simulink model "Quest"  (R2024b)
settings: Solver=VariableStepAuto  StartTime=0.0  StopTime=10.0  RelTol=1e-3
libraries: matrix_library x2
settings Model: Creator=parrot  LastModifiedBy=parrot

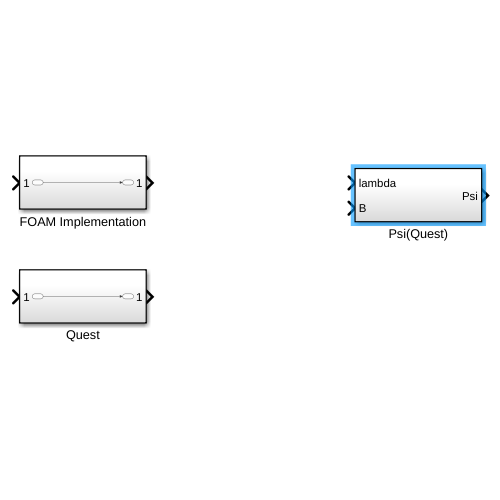
[thumbnail: Simulink's stored preview of the top-level diagram]
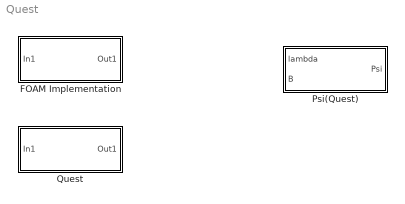
== system Quest ==
  FOAM Implementation : Subsystem
  Psi(Quest) : Subsystem
  Quest : Subsystem

== system Quest/FOAM Implementation ==
  In1 : Inport
  Out1 : Outport
  wires:
  In1/1 -> Out1/1

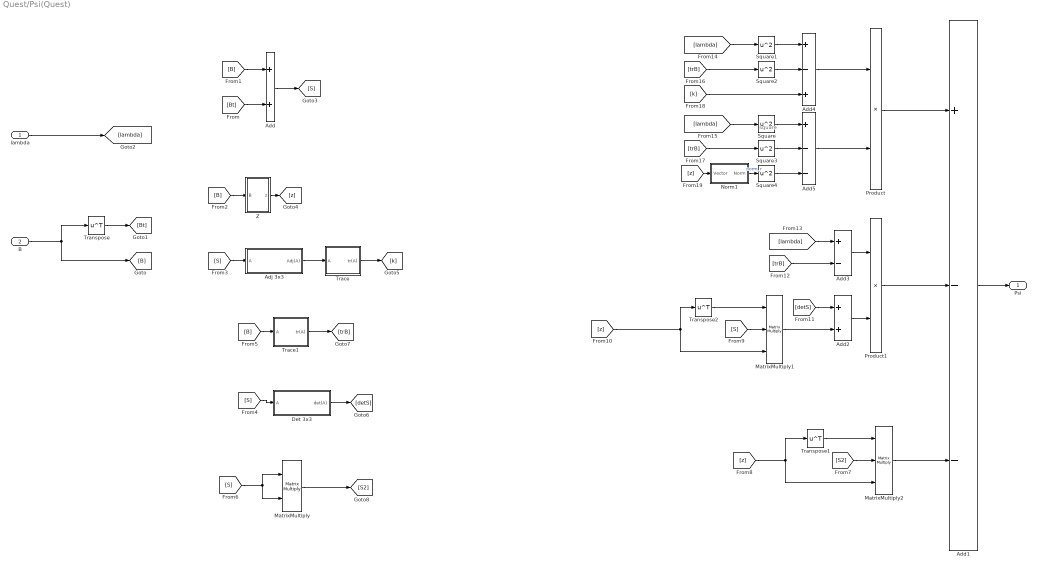
== system Quest/Psi(Quest) ==
  note: square
  lambda : Inport
  B : Inport  Port=2
  Add : Sum
  Add1 : Sum  Inputs=+--
  Add2 : Sum
  Add3 : Sum  Inputs=+-
  Add4 : Sum  Inputs=+-+
  Add5 : Sum  Inputs=+--
  Adj 3x3 : Subsystem
  Det 3x3 : Subsystem
  MatrixMultiply : Product  Multiplication=Matrix(*)
  MatrixMultiply1 : Product  Inputs=3  Multiplication=Matrix(*)
  MatrixMultiply2 : Product  Inputs=3  Multiplication=Matrix(*)
  Norm1 : Subsystem
  Product : Product
  Product1 : Product
  Square{,1..4} (5 alike) : Math  Operator=square
  Trace : Subsystem
  Trace1 : Subsystem
  Transpose : Math  Operator=transpose
  Transpose1 : Math  Operator=transpose
  Transpose2 : Math  Operator=transpose
  Z : Subsystem
  Psi : Outport
  wires:
  Transpose/1 -> [Bt]
  B/1 -> Transpose/1, [B]
  lambda/1 -> [lambda]
  Add/1 -> [S]
  [B] -> Add/1
  [Bt] -> Add/2
  Z/1(z) -> [z]
  [B] -> Z/1(B)
  Adj 3x3/1(Adj(A)) -> Trace/1(A)
  Trace/1(tr(A)) -> [k]
  [S] -> Adj 3x3/1(A)
  [S] -> Det 3x3/1(A)
  Det 3x3/1(det(A)) -> [detS]
  [B] -> Trace1/1(A)
  Trace1/1(tr(A)) -> [trB]
  Add1/1 -> Psi/1
  Product/1 -> Add1/1
  Product1/1 -> Add1/2
  [S] -> MatrixMultiply/1, MatrixMultiply/2
  MatrixMultiply/1 -> [S2]
  MatrixMultiply2/1 -> Add1/3
  [S2] -> MatrixMultiply2/2
  Transpose1/1 -> MatrixMultiply2/1
  [z] -> MatrixMultiply2/3, Transpose1/1
  Transpose2/1 -> MatrixMultiply1/1
  [S] -> MatrixMultiply1/2
  [z] -> MatrixMultiply1/3, Transpose2/1
  Add2/1 -> Product1/2
  MatrixMultiply1/1 -> Add2/2
  [detS] -> Add2/1
  Add3/1 -> Product1/1
  [trB] -> Add3/2
  [lambda] -> Add3/1
  Add4/1 -> Product/1
  Add5/1 -> Product/2
  Square/1 -> Add5/1
  Square1/1 -> Add4/1
  [lambda] -> Square1/1
  [lambda] -> Square/1
  Square2/1 -> Add4/2
  Square3/1 -> Add5/2
  [trB] -> Square2/1
  [trB] -> Square3/1
  Square4/1 -> Add5/3
  [k] -> Add4/3
  Norm1/1(Norm) -> Square4/1  "norm_r"
  [z] -> Norm1/1(Vector)

== system Quest/Quest ==
  In1 : Inport
  Out1 : Outport
  wires:
  In1/1 -> Out1/1

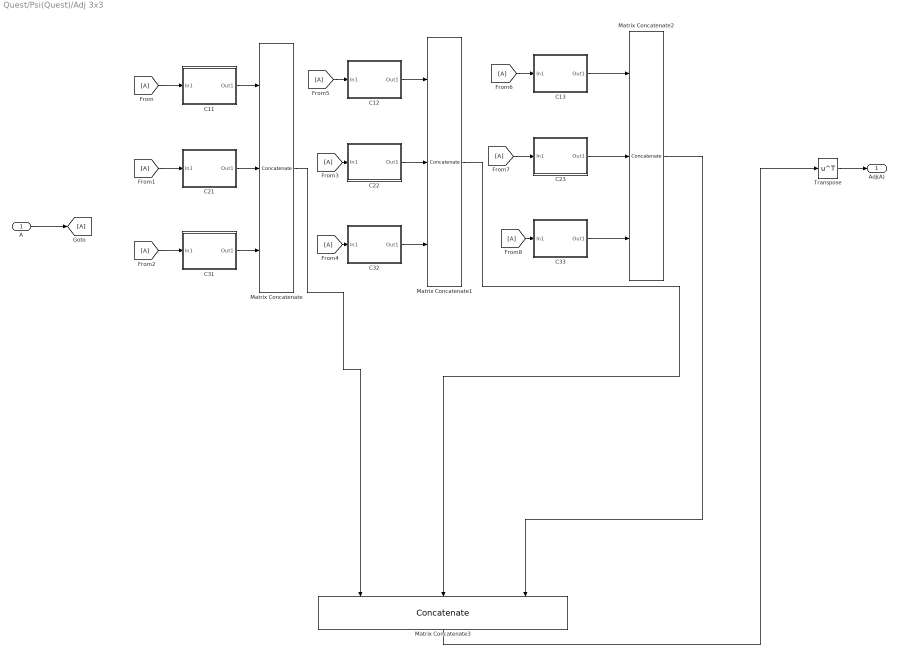
== system Quest/Psi(Quest)/Adj 3x3 ==
  A : Inport
  C11 : Subsystem
  C12 : Subsystem
  C13 : Subsystem
  C21 : Subsystem
  C22 : Subsystem
  C23 : Subsystem
  C31 : Subsystem
  C32 : Subsystem
  C33 : Subsystem
  From{,1..8} (9 alike) : From
  Goto : Goto
  Matrix Concatenate : Concatenate  NumInputs=3  Mode=Multidimensional array
  Matrix Concatenate1 : Concatenate  NumInputs=3  Mode=Multidimensional array
  Matrix Concatenate2 : Concatenate  NumInputs=3  Mode=Multidimensional array
  Matrix Concatenate3 : Concatenate  NumInputs=3  Mode=Multidimensional array  ConcatenateDimension=2
  Transpose : Math  Operator=transpose
  Adj(A) : Outport
  wires:
  Transpose/1 -> Adj(A)/1
  A/1 -> Goto/1
  C11/1(Out1) -> Matrix Concatenate/1
  C21/1(Out1) -> Matrix Concatenate/2
  C31/1(Out1) -> Matrix Concatenate/3
  C22/1(Out1) -> Matrix Concatenate1/2
  C12/1(Out1) -> Matrix Concatenate1/1
  C32/1(Out1) -> Matrix Concatenate1/3
  C23/1(Out1) -> Matrix Concatenate2/2
  C13/1(Out1) -> Matrix Concatenate2/1
  C33/1(Out1) -> Matrix Concatenate2/3
  Matrix Concatenate3/1 -> Transpose/1
  Matrix Concatenate2/1 -> Matrix Concatenate3/3
  Matrix Concatenate1/1 -> Matrix Concatenate3/2
  Matrix Concatenate/1 -> Matrix Concatenate3/1
  From/1 -> C11/1(In1)
  From1/1 -> C21/1(In1)
  From2/1 -> C31/1(In1)
  From3/1 -> C22/1(In1)
  From4/1 -> C32/1(In1)
  From5/1 -> C12/1(In1)
  From6/1 -> C13/1(In1)
  From7/1 -> C23/1(In1)
  From8/1 -> C33/1(In1)

== system Quest/Psi(Quest)/Det 3x3 ==
  A : Inport
  Adj 3x3 : Subsystem
  Matrix Multiply : Product  Multiplication=Matrix(*)
  Selector : Selector  NumberOfDimensions=2  InputPortWidth=3  IndexOptions=Index vector (dialog),Index vector (dialog)  Indices=1,1  OutputSizes=1,1
  det(A) : Outport
  wires:
  A/1 -> Adj 3x3/1(In1), Matrix Multiply/1
  Adj 3x3/1(Out1) -> Matrix Multiply/2
  Matrix Multiply/1 -> Selector/1
  Selector/1 -> det(A)/1

== system Quest/Psi(Quest)/Norm1 ==
  Vector : Inport
  Add : Sum  Inputs=+++
  Demux : Demux  Outputs=3
  Sqrt : Sqrt
  Square : Math  Operator=square
  Square1 : Math  Operator=square
  Square2 : Math  Operator=square
  Norm : Outport
  wires:
  Square/1 -> Add/1
  Add/1 -> Sqrt/1
  Demux/3 -> Square1/1
  Square2/1 -> Add/2
  Square1/1 -> Add/3
  Demux/1 -> Square/1
  Demux/2 -> Square2/1
  Vector/1 -> Demux/1
  Sqrt/1 -> Norm/1

== system Quest/Psi(Quest)/Trace ==
  A : Inport
  Extract Diagonal : matrix_library/Extract Diagonal
      settings: LibrarySourceBlock=|
      | simulink/Matrix
      | Operations/Extract Diagonal
  Sum of Elements : Sum  Inputs=+
  tr(A) : Outport
  wires:
  A/1 -> Extract Diagonal/1
  Extract Diagonal/1 -> Sum of Elements/1
  Sum of Elements/1 -> tr(A)/1

== system Quest/Psi(Quest)/Trace1 ==
  A : Inport
  Extract Diagonal : matrix_library/Extract Diagonal
  Sum of Elements : Sum  Inputs=+
  tr(A) : Outport
  wires:
  A/1 -> Extract Diagonal/1
  Extract Diagonal/1 -> Sum of Elements/1
  Sum of Elements/1 -> tr(A)/1

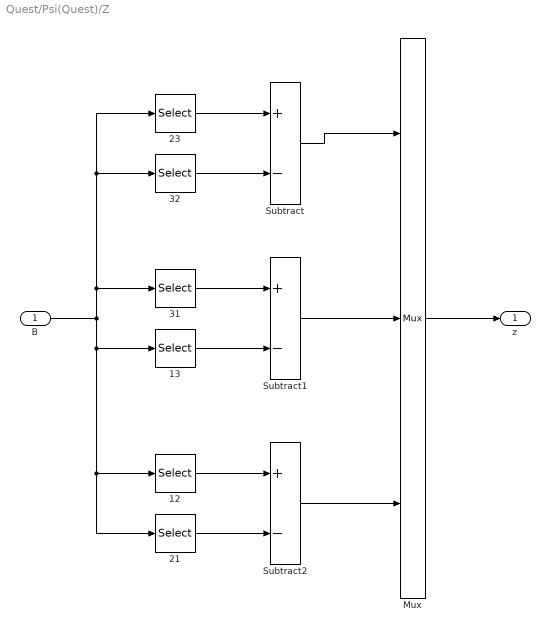
== system Quest/Psi(Quest)/Z ==
  B : Inport
  12 : Selector  NumberOfDimensions=2  InputPortWidth=3  IndexOptions=Index vector (dialog),Index vector (dialog)  Indices=1,2  OutputSizes=1,1
  13 : Selector  NumberOfDimensions=2  InputPortWidth=3  IndexOptions=Index vector (dialog),Index vector (dialog)  Indices=1,3  OutputSizes=1,1
  21 : Selector  NumberOfDimensions=2  InputPortWidth=3  IndexOptions=Index vector (dialog),Index vector (dialog)  Indices=2,1  OutputSizes=1,1
  23 : Selector  NumberOfDimensions=2  InputPortWidth=3  IndexOptions=Index vector (dialog),Index vector (dialog)  Indices=2,3  OutputSizes=1,1
  31 : Selector  NumberOfDimensions=2  InputPortWidth=3  IndexOptions=Index vector (dialog),Index vector (dialog)  Indices=3,1  OutputSizes=1,1
  32 : Selector  NumberOfDimensions=2  InputPortWidth=3  IndexOptions=Index vector (dialog),Index vector (dialog)  Indices=3,2  OutputSizes=1,1
  Mux : Mux  Inputs=3
  Subtract : Sum  Inputs=+-
  Subtract1 : Sum  Inputs=+-
  Subtract2 : Sum  Inputs=+-
  z : Outport
  wires:
  Subtract1/1 -> Mux/2
  31/1 -> Subtract1/1
  Subtract/1 -> Mux/1
  Mux/1 -> z/1
  13/1 -> Subtract1/2
  32/1 -> Subtract/2
  12/1 -> Subtract2/1
  23/1 -> Subtract/1
  Subtract2/1 -> Mux/3
  B/1 -> 31/1, 32/1, 23/1, 13/1, 12/1, 21/1
  21/1 -> Subtract2/2

== system Quest/Psi(Quest)/Adj 3x3/C11 ==
  In1 : Inport
  22 : Selector  NumberOfDimensions=2  InputPortWidth=3  IndexOptions=Index vector (dialog),Index vector (dialog)  Indices=2,2  OutputSizes=1,1
  23 : Selector  NumberOfDimensions=2  InputPortWidth=3  IndexOptions=Index vector (dialog),Index vector (dialog)  Indices=2,3  OutputSizes=1,1
  32 : Selector  NumberOfDimensions=2  InputPortWidth=3  IndexOptions=Index vector (dialog),Index vector (dialog)  Indices=3,2  OutputSizes=1,1
  33 : Selector  NumberOfDimensions=2  InputPortWidth=3  IndexOptions=Index vector (dialog),Index vector (dialog)  Indices=3,3  OutputSizes=1,1
  Product : Product
  Product1 : Product
  Subtract : Sum  Inputs=+-
  Out1 : Outport
  wires:
  In1/1 -> 32/1, 23/1, 33/1, 22/1
  22/1 -> Product/1
  33/1 -> Product/2
  23/1 -> Product1/1
  32/1 -> Product1/2
  Subtract/1 -> Out1/1
  Product/1 -> Subtract/1
  Product1/1 -> Subtract/2

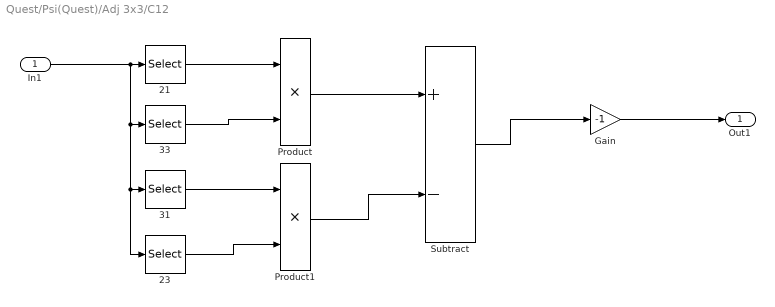
== system Quest/Psi(Quest)/Adj 3x3/C12 ==
  In1 : Inport
  21 : Selector  NumberOfDimensions=2  InputPortWidth=3  IndexOptions=Index vector (dialog),Index vector (dialog)  Indices=2,1  OutputSizes=1,1
  23 : Selector  NumberOfDimensions=2  InputPortWidth=3  IndexOptions=Index vector (dialog),Index vector (dialog)  Indices=2,3  OutputSizes=1,1
  31 : Selector  NumberOfDimensions=2  InputPortWidth=3  IndexOptions=Index vector (dialog),Index vector (dialog)  Indices=3,1  OutputSizes=1,1
  33 : Selector  NumberOfDimensions=2  InputPortWidth=3  IndexOptions=Index vector (dialog),Index vector (dialog)  Indices=3,3  OutputSizes=1,1
  Gain : Gain  Gain=-1
  Product : Product
  Product1 : Product
  Subtract : Sum  Inputs=+-
  Out1 : Outport
  wires:
  In1/1 -> 23/1, 31/1, 33/1, 21/1
  21/1 -> Product/1
  33/1 -> Product/2
  31/1 -> Product1/1
  23/1 -> Product1/2
  Subtract/1 -> Gain/1
  Product/1 -> Subtract/1
  Product1/1 -> Subtract/2
  Gain/1 -> Out1/1

== system Quest/Psi(Quest)/Adj 3x3/C13 ==
  In1 : Inport
  21 : Selector  NumberOfDimensions=2  InputPortWidth=3  IndexOptions=Index vector (dialog),Index vector (dialog)  Indices=2,1  OutputSizes=1,1
  22 : Selector  NumberOfDimensions=2  InputPortWidth=3  IndexOptions=Index vector (dialog),Index vector (dialog)  Indices=2,2  OutputSizes=1,1
  31 : Selector  NumberOfDimensions=2  InputPortWidth=3  IndexOptions=Index vector (dialog),Index vector (dialog)  Indices=3,1  OutputSizes=1,1
  32 : Selector  NumberOfDimensions=2  InputPortWidth=3  IndexOptions=Index vector (dialog),Index vector (dialog)  Indices=3,2  OutputSizes=1,1
  Product : Product
  Product1 : Product
  Subtract : Sum  Inputs=+-
  Out1 : Outport
  wires:
  In1/1 -> 31/1, 22/1, 32/1, 21/1
  21/1 -> Product/1
  32/1 -> Product/2
  22/1 -> Product1/1
  31/1 -> Product1/2
  Subtract/1 -> Out1/1
  Product/1 -> Subtract/1
  Product1/1 -> Subtract/2

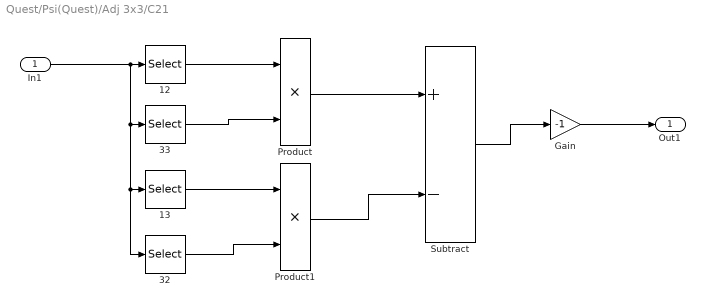
== system Quest/Psi(Quest)/Adj 3x3/C21 ==
  In1 : Inport
  12 : Selector  NumberOfDimensions=2  InputPortWidth=3  IndexOptions=Index vector (dialog),Index vector (dialog)  Indices=1,2  OutputSizes=1,1
  13 : Selector  NumberOfDimensions=2  InputPortWidth=3  IndexOptions=Index vector (dialog),Index vector (dialog)  Indices=1,3  OutputSizes=1,1
  32 : Selector  NumberOfDimensions=2  InputPortWidth=3  IndexOptions=Index vector (dialog),Index vector (dialog)  Indices=3,2  OutputSizes=1,1
  33 : Selector  NumberOfDimensions=2  InputPortWidth=3  IndexOptions=Index vector (dialog),Index vector (dialog)  Indices=3,3  OutputSizes=1,1
  Gain : Gain  Gain=-1
  Product : Product
  Product1 : Product
  Subtract : Sum  Inputs=+-
  Out1 : Outport
  wires:
  In1/1 -> 32/1, 13/1, 33/1, 12/1
  12/1 -> Product/1
  33/1 -> Product/2
  13/1 -> Product1/1
  32/1 -> Product1/2
  Subtract/1 -> Gain/1
  Product/1 -> Subtract/1
  Product1/1 -> Subtract/2
  Gain/1 -> Out1/1

== system Quest/Psi(Quest)/Adj 3x3/C22 ==
  In1 : Inport
  11 : Selector  NumberOfDimensions=2  InputPortWidth=3  IndexOptions=Index vector (dialog),Index vector (dialog)  Indices=1,1  OutputSizes=1,1
  13 : Selector  NumberOfDimensions=2  InputPortWidth=3  IndexOptions=Index vector (dialog),Index vector (dialog)  Indices=1,3  OutputSizes=1,1
  31 : Selector  NumberOfDimensions=2  InputPortWidth=3  IndexOptions=Index vector (dialog),Index vector (dialog)  Indices=3,1  OutputSizes=1,1
  33 : Selector  NumberOfDimensions=2  InputPortWidth=3  IndexOptions=Index vector (dialog),Index vector (dialog)  Indices=3,3  OutputSizes=1,1
  Product : Product
  Product1 : Product
  Subtract : Sum  Inputs=+-
  Out1 : Outport
  wires:
  In1/1 -> 31/1, 13/1, 33/1, 11/1
  11/1 -> Product/1
  33/1 -> Product/2
  13/1 -> Product1/1
  31/1 -> Product1/2
  Subtract/1 -> Out1/1
  Product/1 -> Subtract/1
  Product1/1 -> Subtract/2

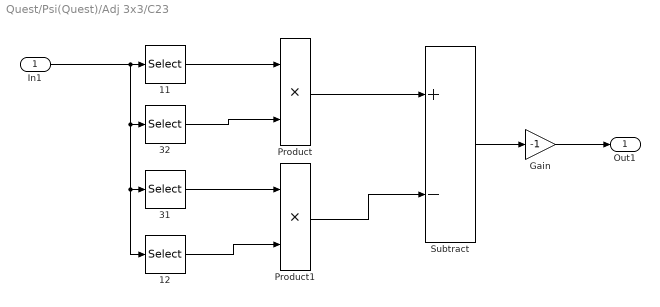
== system Quest/Psi(Quest)/Adj 3x3/C23 ==
  In1 : Inport
  11 : Selector  NumberOfDimensions=2  InputPortWidth=3  IndexOptions=Index vector (dialog),Index vector (dialog)  Indices=1,1  OutputSizes=1,1
  12 : Selector  NumberOfDimensions=2  InputPortWidth=3  IndexOptions=Index vector (dialog),Index vector (dialog)  Indices=1,2  OutputSizes=1,1
  31 : Selector  NumberOfDimensions=2  InputPortWidth=3  IndexOptions=Index vector (dialog),Index vector (dialog)  Indices=3,1  OutputSizes=1,1
  32 : Selector  NumberOfDimensions=2  InputPortWidth=3  IndexOptions=Index vector (dialog),Index vector (dialog)  Indices=3,2  OutputSizes=1,1
  Gain : Gain  Gain=-1
  Product : Product
  Product1 : Product
  Subtract : Sum  Inputs=+-
  Out1 : Outport
  wires:
  In1/1 -> 12/1, 31/1, 32/1, 11/1
  11/1 -> Product/1
  32/1 -> Product/2
  31/1 -> Product1/1
  12/1 -> Product1/2
  Subtract/1 -> Gain/1
  Product/1 -> Subtract/1
  Product1/1 -> Subtract/2
  Gain/1 -> Out1/1

== system Quest/Psi(Quest)/Adj 3x3/C31 ==
  In1 : Inport
  12 : Selector  NumberOfDimensions=2  InputPortWidth=3  IndexOptions=Index vector (dialog),Index vector (dialog)  Indices=1,2  OutputSizes=1,1
  13 : Selector  NumberOfDimensions=2  InputPortWidth=3  IndexOptions=Index vector (dialog),Index vector (dialog)  Indices=1,3  OutputSizes=1,1
  22 : Selector  NumberOfDimensions=2  InputPortWidth=3  IndexOptions=Index vector (dialog),Index vector (dialog)  Indices=2,2  OutputSizes=1,1
  23 : Selector  NumberOfDimensions=2  InputPortWidth=3  IndexOptions=Index vector (dialog),Index vector (dialog)  Indices=2,3  OutputSizes=1,1
  Product : Product
  Product1 : Product
  Subtract : Sum  Inputs=+-
  Out1 : Outport
  wires:
  In1/1 -> 22/1, 13/1, 23/1, 12/1
  12/1 -> Product/1
  23/1 -> Product/2
  13/1 -> Product1/1
  22/1 -> Product1/2
  Subtract/1 -> Out1/1
  Product/1 -> Subtract/1
  Product1/1 -> Subtract/2

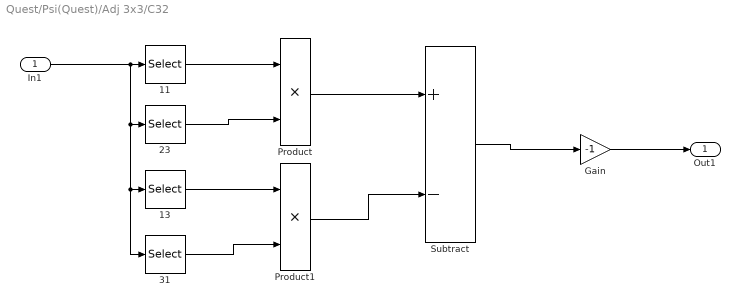
== system Quest/Psi(Quest)/Adj 3x3/C32 ==
  In1 : Inport
  11 : Selector  NumberOfDimensions=2  InputPortWidth=3  IndexOptions=Index vector (dialog),Index vector (dialog)  Indices=1,1  OutputSizes=1,1
  13 : Selector  NumberOfDimensions=2  InputPortWidth=3  IndexOptions=Index vector (dialog),Index vector (dialog)  Indices=1,3  OutputSizes=1,1
  23 : Selector  NumberOfDimensions=2  InputPortWidth=3  IndexOptions=Index vector (dialog),Index vector (dialog)  Indices=2,3  OutputSizes=1,1
  31 : Selector  NumberOfDimensions=2  InputPortWidth=3  IndexOptions=Index vector (dialog),Index vector (dialog)  Indices=3,1  OutputSizes=1,1
  Gain : Gain  Gain=-1
  Product : Product
  Product1 : Product
  Subtract : Sum  Inputs=+-
  Out1 : Outport
  wires:
  In1/1 -> 31/1, 13/1, 23/1, 11/1
  11/1 -> Product/1
  23/1 -> Product/2
  13/1 -> Product1/1
  31/1 -> Product1/2
  Subtract/1 -> Gain/1
  Product/1 -> Subtract/1
  Product1/1 -> Subtract/2
  Gain/1 -> Out1/1

== system Quest/Psi(Quest)/Adj 3x3/C33 ==
  In1 : Inport
  11 : Selector  NumberOfDimensions=2  InputPortWidth=3  IndexOptions=Index vector (dialog),Index vector (dialog)  Indices=1,1  OutputSizes=1,1
  12 : Selector  NumberOfDimensions=2  InputPortWidth=3  IndexOptions=Index vector (dialog),Index vector (dialog)  Indices=1,2  OutputSizes=1,1
  21 : Selector  NumberOfDimensions=2  InputPortWidth=3  IndexOptions=Index vector (dialog),Index vector (dialog)  Indices=2,1  OutputSizes=1,1
  22 : Selector  NumberOfDimensions=2  InputPortWidth=3  IndexOptions=Index vector (dialog),Index vector (dialog)  Indices=2,2  OutputSizes=1,1
  Product : Product
  Product1 : Product
  Subtract : Sum  Inputs=+-
  Out1 : Outport
  wires:
  In1/1 -> 21/1, 12/1, 22/1, 11/1
  11/1 -> Product/1
  22/1 -> Product/2
  12/1 -> Product1/1
  21/1 -> Product1/2
  Subtract/1 -> Out1/1
  Product/1 -> Subtract/1
  Product1/1 -> Subtract/2

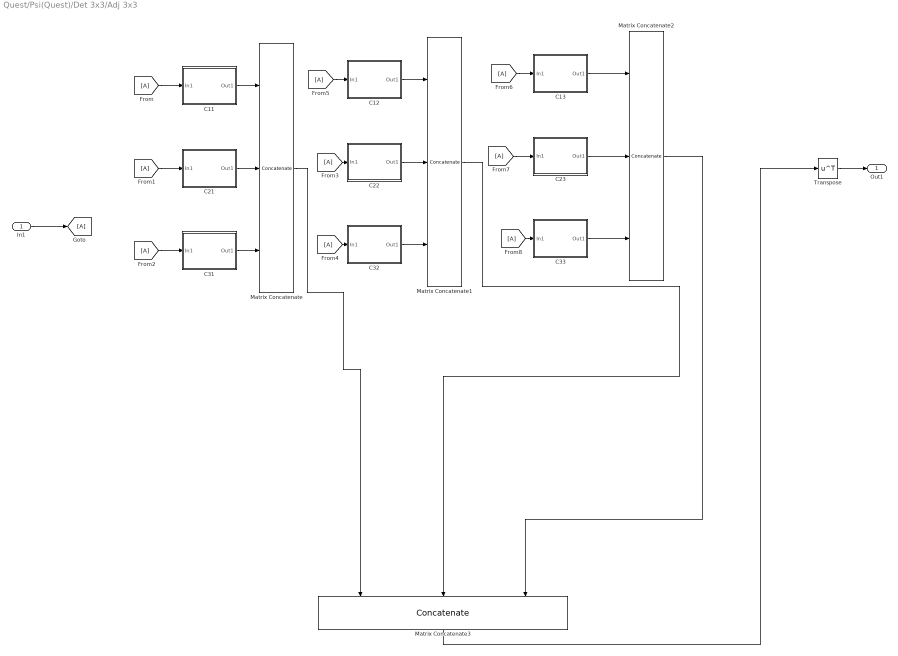
== system Quest/Psi(Quest)/Det 3x3/Adj 3x3 ==
  In1 : Inport
  C11 : Subsystem
  C12 : Subsystem
  C13 : Subsystem
  C21 : Subsystem
  C22 : Subsystem
  C23 : Subsystem
  C31 : Subsystem
  C32 : Subsystem
  C33 : Subsystem
  From{,1..8} (9 alike) : From
  Goto : Goto
  Matrix Concatenate : Concatenate  NumInputs=3  Mode=Multidimensional array
  Matrix Concatenate1 : Concatenate  NumInputs=3  Mode=Multidimensional array
  Matrix Concatenate2 : Concatenate  NumInputs=3  Mode=Multidimensional array
  Matrix Concatenate3 : Concatenate  NumInputs=3  Mode=Multidimensional array  ConcatenateDimension=2
  Transpose : Math  Operator=transpose
  Out1 : Outport
  wires:
  Transpose/1 -> Out1/1
  In1/1 -> Goto/1
  C11/1(Out1) -> Matrix Concatenate/1
  C21/1(Out1) -> Matrix Concatenate/2
  C31/1(Out1) -> Matrix Concatenate/3
  C22/1(Out1) -> Matrix Concatenate1/2
  C12/1(Out1) -> Matrix Concatenate1/1
  C32/1(Out1) -> Matrix Concatenate1/3
  C23/1(Out1) -> Matrix Concatenate2/2
  C13/1(Out1) -> Matrix Concatenate2/1
  C33/1(Out1) -> Matrix Concatenate2/3
  Matrix Concatenate3/1 -> Transpose/1
  Matrix Concatenate2/1 -> Matrix Concatenate3/3
  Matrix Concatenate1/1 -> Matrix Concatenate3/2
  Matrix Concatenate/1 -> Matrix Concatenate3/1
  From/1 -> C11/1(In1)
  From1/1 -> C21/1(In1)
  From2/1 -> C31/1(In1)
  From3/1 -> C22/1(In1)
  From4/1 -> C32/1(In1)
  From5/1 -> C12/1(In1)
  From6/1 -> C13/1(In1)
  From7/1 -> C23/1(In1)
  From8/1 -> C33/1(In1)

== system Quest/Psi(Quest)/Det 3x3/Adj 3x3/C11 ==
  In1 : Inport
  22 : Selector  NumberOfDimensions=2  InputPortWidth=3  IndexOptions=Index vector (dialog),Index vector (dialog)  Indices=2,2  OutputSizes=1,1
  23 : Selector  NumberOfDimensions=2  InputPortWidth=3  IndexOptions=Index vector (dialog),Index vector (dialog)  Indices=2,3  OutputSizes=1,1
  32 : Selector  NumberOfDimensions=2  InputPortWidth=3  IndexOptions=Index vector (dialog),Index vector (dialog)  Indices=3,2  OutputSizes=1,1
  33 : Selector  NumberOfDimensions=2  InputPortWidth=3  IndexOptions=Index vector (dialog),Index vector (dialog)  Indices=3,3  OutputSizes=1,1
  Product : Product
  Product1 : Product
  Subtract : Sum  Inputs=+-
  Out1 : Outport
  wires:
  In1/1 -> 32/1, 23/1, 33/1, 22/1
  22/1 -> Product/1
  33/1 -> Product/2
  23/1 -> Product1/1
  32/1 -> Product1/2
  Subtract/1 -> Out1/1
  Product/1 -> Subtract/1
  Product1/1 -> Subtract/2

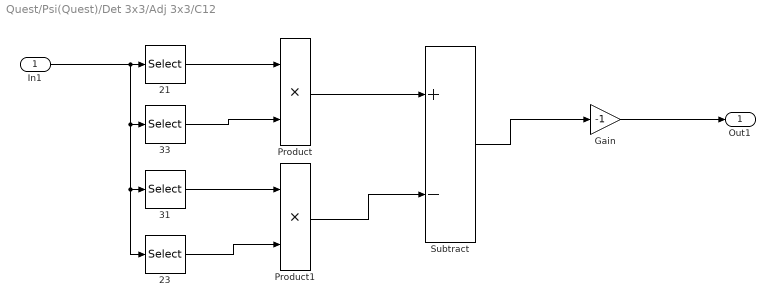
== system Quest/Psi(Quest)/Det 3x3/Adj 3x3/C12 ==
  In1 : Inport
  21 : Selector  NumberOfDimensions=2  InputPortWidth=3  IndexOptions=Index vector (dialog),Index vector (dialog)  Indices=2,1  OutputSizes=1,1
  23 : Selector  NumberOfDimensions=2  InputPortWidth=3  IndexOptions=Index vector (dialog),Index vector (dialog)  Indices=2,3  OutputSizes=1,1
  31 : Selector  NumberOfDimensions=2  InputPortWidth=3  IndexOptions=Index vector (dialog),Index vector (dialog)  Indices=3,1  OutputSizes=1,1
  33 : Selector  NumberOfDimensions=2  InputPortWidth=3  IndexOptions=Index vector (dialog),Index vector (dialog)  Indices=3,3  OutputSizes=1,1
  Gain : Gain  Gain=-1
  Product : Product
  Product1 : Product
  Subtract : Sum  Inputs=+-
  Out1 : Outport
  wires:
  In1/1 -> 23/1, 31/1, 33/1, 21/1
  21/1 -> Product/1
  33/1 -> Product/2
  31/1 -> Product1/1
  23/1 -> Product1/2
  Subtract/1 -> Gain/1
  Product/1 -> Subtract/1
  Product1/1 -> Subtract/2
  Gain/1 -> Out1/1

== system Quest/Psi(Quest)/Det 3x3/Adj 3x3/C13 ==
  In1 : Inport
  21 : Selector  NumberOfDimensions=2  InputPortWidth=3  IndexOptions=Index vector (dialog),Index vector (dialog)  Indices=2,1  OutputSizes=1,1
  22 : Selector  NumberOfDimensions=2  InputPortWidth=3  IndexOptions=Index vector (dialog),Index vector (dialog)  Indices=2,2  OutputSizes=1,1
  31 : Selector  NumberOfDimensions=2  InputPortWidth=3  IndexOptions=Index vector (dialog),Index vector (dialog)  Indices=3,1  OutputSizes=1,1
  32 : Selector  NumberOfDimensions=2  InputPortWidth=3  IndexOptions=Index vector (dialog),Index vector (dialog)  Indices=3,2  OutputSizes=1,1
  Product : Product
  Product1 : Product
  Subtract : Sum  Inputs=+-
  Out1 : Outport
  wires:
  In1/1 -> 31/1, 22/1, 32/1, 21/1
  21/1 -> Product/1
  32/1 -> Product/2
  22/1 -> Product1/1
  31/1 -> Product1/2
  Subtract/1 -> Out1/1
  Product/1 -> Subtract/1
  Product1/1 -> Subtract/2

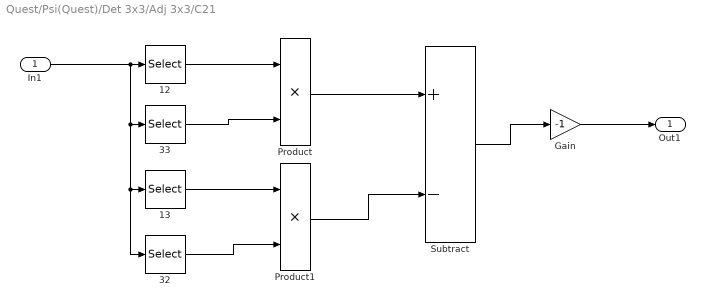
== system Quest/Psi(Quest)/Det 3x3/Adj 3x3/C21 ==
  In1 : Inport
  12 : Selector  NumberOfDimensions=2  InputPortWidth=3  IndexOptions=Index vector (dialog),Index vector (dialog)  Indices=1,2  OutputSizes=1,1
  13 : Selector  NumberOfDimensions=2  InputPortWidth=3  IndexOptions=Index vector (dialog),Index vector (dialog)  Indices=1,3  OutputSizes=1,1
  32 : Selector  NumberOfDimensions=2  InputPortWidth=3  IndexOptions=Index vector (dialog),Index vector (dialog)  Indices=3,2  OutputSizes=1,1
  33 : Selector  NumberOfDimensions=2  InputPortWidth=3  IndexOptions=Index vector (dialog),Index vector (dialog)  Indices=3,3  OutputSizes=1,1
  Gain : Gain  Gain=-1
  Product : Product
  Product1 : Product
  Subtract : Sum  Inputs=+-
  Out1 : Outport
  wires:
  In1/1 -> 32/1, 13/1, 33/1, 12/1
  12/1 -> Product/1
  33/1 -> Product/2
  13/1 -> Product1/1
  32/1 -> Product1/2
  Subtract/1 -> Gain/1
  Product/1 -> Subtract/1
  Product1/1 -> Subtract/2
  Gain/1 -> Out1/1

== system Quest/Psi(Quest)/Det 3x3/Adj 3x3/C22 ==
  In1 : Inport
  11 : Selector  NumberOfDimensions=2  InputPortWidth=3  IndexOptions=Index vector (dialog),Index vector (dialog)  Indices=1,1  OutputSizes=1,1
  13 : Selector  NumberOfDimensions=2  InputPortWidth=3  IndexOptions=Index vector (dialog),Index vector (dialog)  Indices=1,3  OutputSizes=1,1
  31 : Selector  NumberOfDimensions=2  InputPortWidth=3  IndexOptions=Index vector (dialog),Index vector (dialog)  Indices=3,1  OutputSizes=1,1
  33 : Selector  NumberOfDimensions=2  InputPortWidth=3  IndexOptions=Index vector (dialog),Index vector (dialog)  Indices=3,3  OutputSizes=1,1
  Product : Product
  Product1 : Product
  Subtract : Sum  Inputs=+-
  Out1 : Outport
  wires:
  In1/1 -> 31/1, 13/1, 33/1, 11/1
  11/1 -> Product/1
  33/1 -> Product/2
  13/1 -> Product1/1
  31/1 -> Product1/2
  Subtract/1 -> Out1/1
  Product/1 -> Subtract/1
  Product1/1 -> Subtract/2

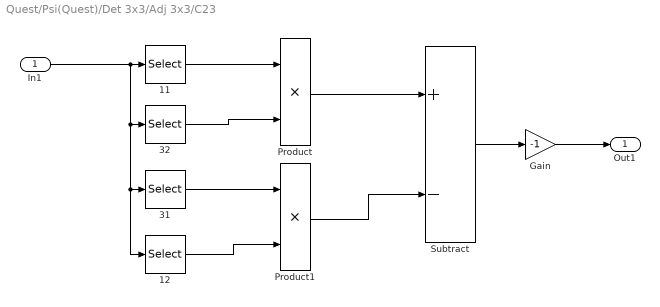
== system Quest/Psi(Quest)/Det 3x3/Adj 3x3/C23 ==
  In1 : Inport
  11 : Selector  NumberOfDimensions=2  InputPortWidth=3  IndexOptions=Index vector (dialog),Index vector (dialog)  Indices=1,1  OutputSizes=1,1
  12 : Selector  NumberOfDimensions=2  InputPortWidth=3  IndexOptions=Index vector (dialog),Index vector (dialog)  Indices=1,2  OutputSizes=1,1
  31 : Selector  NumberOfDimensions=2  InputPortWidth=3  IndexOptions=Index vector (dialog),Index vector (dialog)  Indices=3,1  OutputSizes=1,1
  32 : Selector  NumberOfDimensions=2  InputPortWidth=3  IndexOptions=Index vector (dialog),Index vector (dialog)  Indices=3,2  OutputSizes=1,1
  Gain : Gain  Gain=-1
  Product : Product
  Product1 : Product
  Subtract : Sum  Inputs=+-
  Out1 : Outport
  wires:
  In1/1 -> 12/1, 31/1, 32/1, 11/1
  11/1 -> Product/1
  32/1 -> Product/2
  31/1 -> Product1/1
  12/1 -> Product1/2
  Subtract/1 -> Gain/1
  Product/1 -> Subtract/1
  Product1/1 -> Subtract/2
  Gain/1 -> Out1/1

== system Quest/Psi(Quest)/Det 3x3/Adj 3x3/C31 ==
  In1 : Inport
  12 : Selector  NumberOfDimensions=2  InputPortWidth=3  IndexOptions=Index vector (dialog),Index vector (dialog)  Indices=1,2  OutputSizes=1,1
  13 : Selector  NumberOfDimensions=2  InputPortWidth=3  IndexOptions=Index vector (dialog),Index vector (dialog)  Indices=1,3  OutputSizes=1,1
  22 : Selector  NumberOfDimensions=2  InputPortWidth=3  IndexOptions=Index vector (dialog),Index vector (dialog)  Indices=2,2  OutputSizes=1,1
  23 : Selector  NumberOfDimensions=2  InputPortWidth=3  IndexOptions=Index vector (dialog),Index vector (dialog)  Indices=2,3  OutputSizes=1,1
  Product : Product
  Product1 : Product
  Subtract : Sum  Inputs=+-
  Out1 : Outport
  wires:
  In1/1 -> 22/1, 13/1, 23/1, 12/1
  12/1 -> Product/1
  23/1 -> Product/2
  13/1 -> Product1/1
  22/1 -> Product1/2
  Subtract/1 -> Out1/1
  Product/1 -> Subtract/1
  Product1/1 -> Subtract/2

== system Quest/Psi(Quest)/Det 3x3/Adj 3x3/C32 ==
  In1 : Inport
  11 : Selector  NumberOfDimensions=2  InputPortWidth=3  IndexOptions=Index vector (dialog),Index vector (dialog)  Indices=1,1  OutputSizes=1,1
  13 : Selector  NumberOfDimensions=2  InputPortWidth=3  IndexOptions=Index vector (dialog),Index vector (dialog)  Indices=1,3  OutputSizes=1,1
  23 : Selector  NumberOfDimensions=2  InputPortWidth=3  IndexOptions=Index vector (dialog),Index vector (dialog)  Indices=2,3  OutputSizes=1,1
  31 : Selector  NumberOfDimensions=2  InputPortWidth=3  IndexOptions=Index vector (dialog),Index vector (dialog)  Indices=3,1  OutputSizes=1,1
  Gain : Gain  Gain=-1
  Product : Product
  Product1 : Product
  Subtract : Sum  Inputs=+-
  Out1 : Outport
  wires:
  In1/1 -> 31/1, 13/1, 23/1, 11/1
  11/1 -> Product/1
  23/1 -> Product/2
  13/1 -> Product1/1
  31/1 -> Product1/2
  Subtract/1 -> Gain/1
  Product/1 -> Subtract/1
  Product1/1 -> Subtract/2
  Gain/1 -> Out1/1

== system Quest/Psi(Quest)/Det 3x3/Adj 3x3/C33 ==
  In1 : Inport
  11 : Selector  NumberOfDimensions=2  InputPortWidth=3  IndexOptions=Index vector (dialog),Index vector (dialog)  Indices=1,1  OutputSizes=1,1
  12 : Selector  NumberOfDimensions=2  InputPortWidth=3  IndexOptions=Index vector (dialog),Index vector (dialog)  Indices=1,2  OutputSizes=1,1
  21 : Selector  NumberOfDimensions=2  InputPortWidth=3  IndexOptions=Index vector (dialog),Index vector (dialog)  Indices=2,1  OutputSizes=1,1
  22 : Selector  NumberOfDimensions=2  InputPortWidth=3  IndexOptions=Index vector (dialog),Index vector (dialog)  Indices=2,2  OutputSizes=1,1
  Product : Product
  Product1 : Product
  Subtract : Sum  Inputs=+-
  Out1 : Outport
  wires:
  In1/1 -> 21/1, 12/1, 22/1, 11/1
  11/1 -> Product/1
  22/1 -> Product/2
  12/1 -> Product1/1
  21/1 -> Product1/2
  Subtract/1 -> Out1/1
  Product/1 -> Subtract/1
  Product1/1 -> Subtract/2
